simulink model "hezhiqiang"  (R2014a)
settings: Solver=ode45  StartTime=0.0  StopTime=10.0  RelTol=1e-3
settings Model: Creator=xujiahong  LastModifiedBy=Administrator

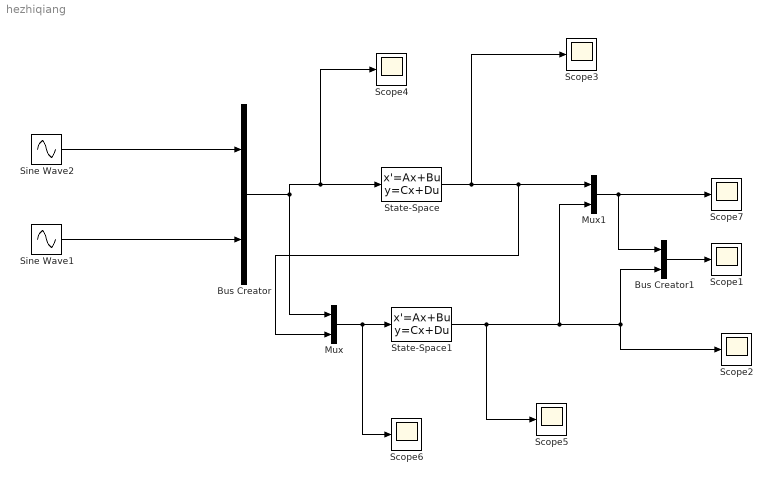
== system hezhiqiang ==
  Bus Creator : BusCreator  Inputs=2
  Bus Creator1 : BusCreator  Inputs=2
  Mux : Mux  Inputs=2
  Mux1 : Mux  Inputs=2
  Scope{1..7} (7 alike) : Scope
      Scope1 settings: SaveName=ScopeData2
      Scope2 settings: SaveName=ScopeData3
      Scope3 settings: SaveName=ScopeData4
      Scope4 settings: SaveName=ScopeData5
      Scope6 settings: SaveName=ScopeData6
      Scope7 settings: SaveName=ScopeData7
  Sine Wave1 : Sin  Frequency=5  Phase=0.5*pi  SampleTime=0
  Sine Wave2 : Sin  Frequency=5  SampleTime=0
  State-Space : StateSpace  A=[-110.2424 0 200.9966 0;0 -110.2424 0 200.9966;107.1489 0 -206.7995 0;0 107.1489 0 -206.7995]  B=[253.4307 0;0 253.4307;-264.3194 0;0 -246.3194]  C=[1 0 0 0;0 1 0 0]  D=[0 0;0 0]  X0=[0 0 0 0]
  State-Space1 : StateSpace  A=[-110.2424 0 200.9966 0;0 -110.2424 0 200.9966;107.1489 0 -206.7995 0;0 107.1489 0 -206.7995]-[-44.8158 -22.9369;52.4034 -97.3340;79.4732 -8.2236;-6.9857 129.4281]*[1 0 0 0;0 1 0 0]  B=[[253.4307 0;0 253.4307;-264.3194 0;0 -246.3194]-[-44.8158 -22.9369;52.4034 -97.3340;79.4732 -8.2236;-6.9857 129.4281]*[0 0;0 0] [-44.8158 -22.9369;52.4034 -97.3340;79.4732 -8.2236;-6.9857 129.4281]]  C=[1 0 0 0;0 1 0 0]  D=[0 0 0 0;0 0 0 0]  X0=[0.51 0.5 0.5 0.5]
  wires:
  State-Space/1 -> Mux/2, Mux1/1, Scope3/1
  Mux/1 -> Scope6/1, State-Space1/1
  Bus Creator1/1 -> Scope1/1
  Mux1/1 -> Scope7/1, Bus Creator1/1
  State-Space1/1 -> Scope5/1, Mux1/2, Scope2/1, Bus Creator1/2
  Bus Creator/1 -> Scope4/1, State-Space/1, Mux/1
  Sine Wave1/1 -> Bus Creator/2
  Sine Wave2/1 -> Bus Creator/1
